simulink model "EV_Main_Model"  (R2024b)
settings: Solver=VariableStepAuto  StartTime=0.0  StopTime=10.0  RelTol=1e-3
settings Model: Creator=HP ELITEBOOK  LastModifiedBy=HP ELITEBOOK

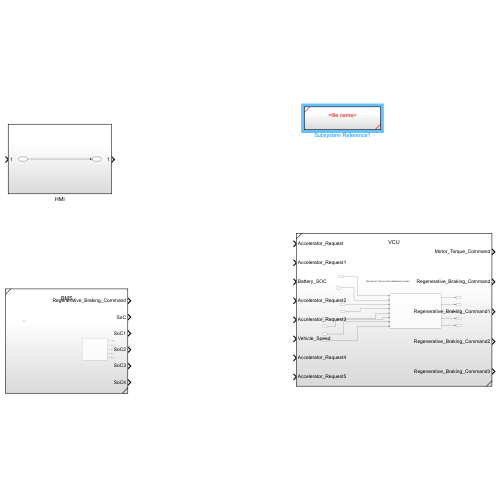
[thumbnail: Simulink's stored preview of the top-level diagram]
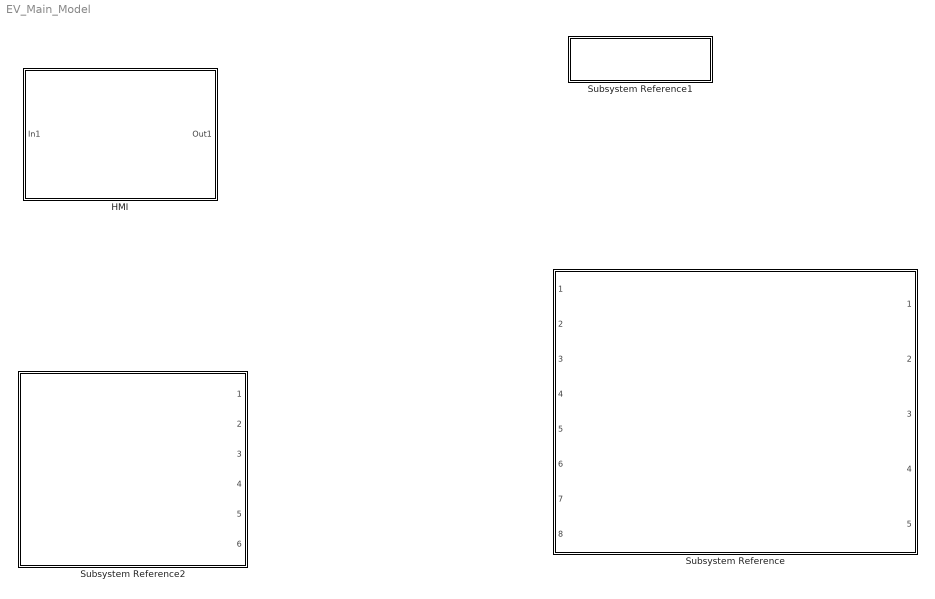
== system EV_Main_Model ==
  HMI : Subsystem
  Subsystem Reference : Subsystem  ReferencedSubsystem=VCU
  Subsystem Reference1 : Subsystem  ReferencedSubsystem=<file name>
  Subsystem Reference2 : Subsystem  ReferencedSubsystem=BMS

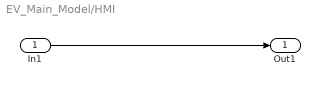
== system EV_Main_Model/HMI ==
  In1 : Inport
  Out1 : Outport
  wires:
  In1/1 -> Out1/1

== system EV_Main_Model/Subsystem Reference1 ==
